simulink model "Szakdoga"  (R2018a)
settings: Solver=ode23s  StartTime=0.0  StopTime=6  RelTol=1e-3
values from neighbouring files (symbols this model uses):
  alp1 = (m1*lc1^2) + (m2*(l1^2+lc2^2)+I1+I2)    (= 1.6375)    [variables.m]
  alp2 = m2*l1*lc2    (= 0.4)    [variables.m]
  alp3 = (m2*lc2^2) + I2    (= 0.216667)    [variables.m]
undefined symbols (not defined in the file or in its folder): DiscIntNeverNeededParam
libraries: nesl_utility x9, sm_lib x8, simulink x6
settings Model: Creator=cloud  LastModifiedBy=cloud

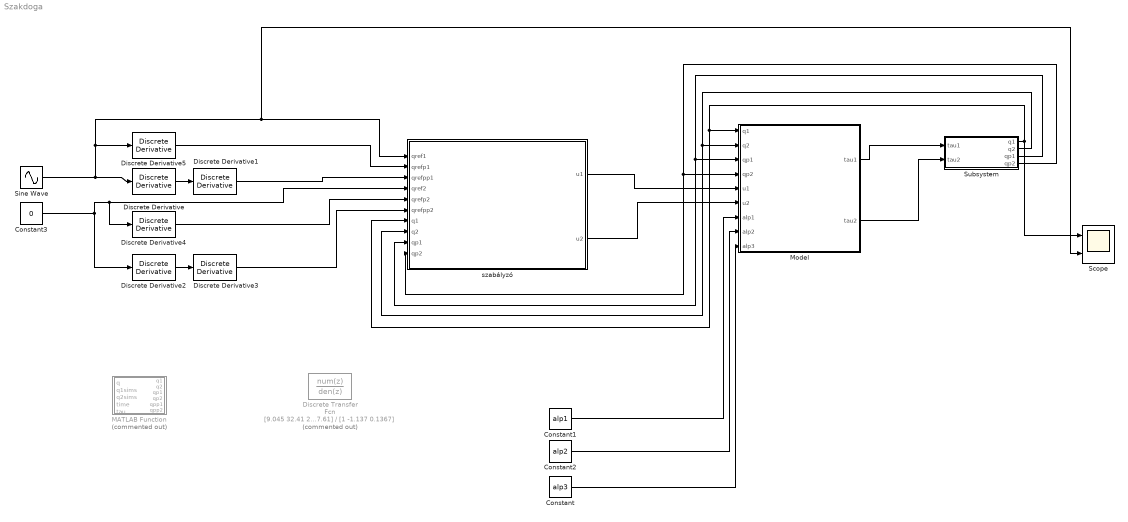
== system Szakdoga ==
  Constant : Constant  Value=alp3
  Constant1 : Constant  Value=alp1
  Constant2 : Constant  Value=alp2
  Constant3 : Constant  Value=0
  Discrete Transfer Fcn : DiscreteTransferFcn  Commented=on  Numerator=[9.045 32.41 27.61]  Denominator=[1 -1.137 0.1367]
  Discrete Derivative{,1..5} (6 alike) : simulink/Discrete/Discrete Derivative  gainval=1.0  ICPrevScaledInput=0.0  OutMin=[]  OutMax=[]  OutDataType=fixdt(1, 16)  OutScaling=2^-10  DoSatur=off
  MATLAB Function : MATLAB Function  Commented=on  TreatAsAtomicUnit=on
  Model : MATLAB Function  TreatAsAtomicUnit=on
  Scope : Scope  NumInputPorts=2
  Sine Wave : Sin  Amplitude=pi/2  Bias=pi/2  Frequency=1.5  SampleTime=0
  Subsystem : Subsystem
  szabályzó : Subsystem
  wires:
  Model/2(tau2) -> Subsystem/2(tau2)
  Model/1(tau1) -> Subsystem/1(tau1)
  Subsystem/2(q2) -> Model/2(q2), szabályzó/8(q2)
  Subsystem/3(qp1) -> Model/3(qp1), szabályzó/9(qp1)
  Subsystem/4(qp2) -> szabályzó/10(qp2), Model/4(qp2)
  Sine Wave/1 -> Discrete Derivative/1, Discrete Derivative5/1, Scope/2, szabályzó/1(qref1)
  Constant3/1 -> szabályzó/4(qref2), Discrete Derivative4/1, Discrete Derivative2/1
  Constant/1 -> Model/9(alp3)
  Constant2/1 -> Model/8(alp2)
  Constant1/1 -> Model/7(alp1)
  Discrete Derivative/1 -> Discrete Derivative1/1
  Discrete Derivative5/1 -> szabályzó/2(qrefp1)
  Discrete Derivative1/1 -> szabályzó/3(qrefpp1)
  Discrete Derivative4/1 -> szabályzó/5(qrefp2)
  szabályzó/1(u1) -> Model/5(u1)
  szabályzó/2(u2) -> Model/6(u2)
  Subsystem/1("q1 ") -> szabályzó/7(q1), Model/1(q1), Scope/1
  Discrete Derivative2/1 -> Discrete Derivative3/1
  Discrete Derivative3/1 -> szabályzó/6(qrefpp2)

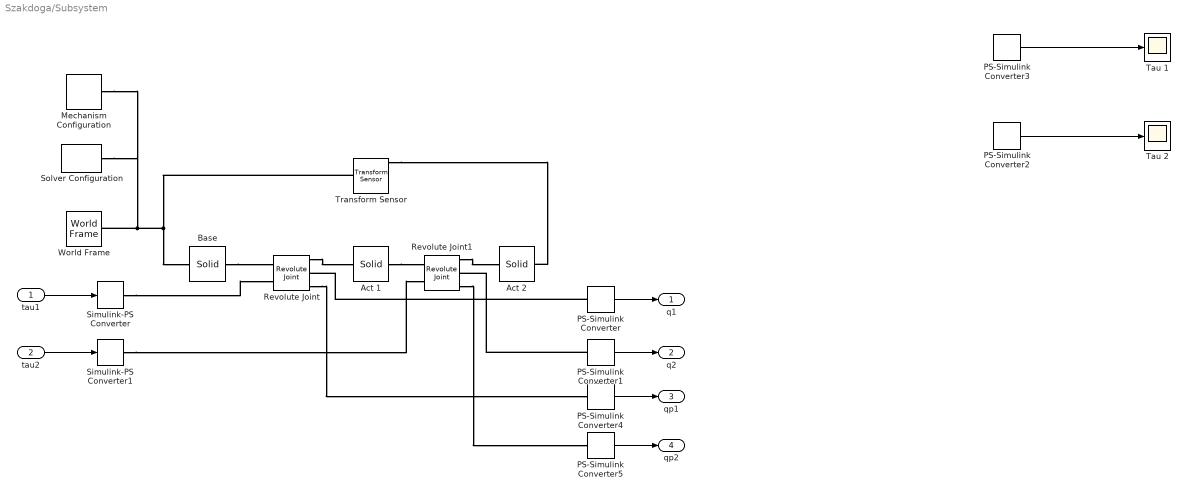
== system Szakdoga/Subsystem ==
  tau1 : Inport
  tau2 : Inport  Port=2
  Act 1 : sm_lib/Body Elements/Solid  InertiaType=CalculateFromGeometry  Mass=1  MassUnits=kg  CenterOfMass=[0 0 0]  CenterOfMassUnits=m  MomentsOfInertia=[1 1 1]  MomentsOfInertiaUnits=kg*m^2  ProductsOfInertia=[0 0 0]  ProductsOfInertiaUnits=kg*m^2  DensityBased=on  Density=1000  DensityUnits=kg/m^3  DoExposeReferenceFrame=off  SerializedFrames=<Frames><Frame><Id>Frame1</Id><Value><Name>F1</Name><Origin><Source>GeometricFeature</Source><FeatureName>-y -z curve</FeatureName></Origin><PrimaryAxis><DefinedDirection>+Z</DefinedDirection><Source>ReferenceFrame</Source><SourceDirection>+Z</SourceDirection><FeatureName></FeatureName></PrimaryAxis><SecondaryAxis><DefinedDirection>+X</DefinedDirection><Source>ReferenceFrame</Source><SourceDirection>+X</SourceDirection><FeatureName></FeatureName></SecondaryAxis></Value></Frame><Frame><Id>Frame2</Id><Value><Name>F2</Name><Origin><Source>GeometricFeature</Source><FeatureName>+y -z curve</FeatureName></Origin><PrimaryAxis><DefinedDirection>+Z</DefinedDirection><Source>ReferenceFrame</Source><SourceDirection>+Z</SourceDirection><FeatureName></FeatureName></PrimaryAxis><SecondaryAxis><DefinedDirection>+X</DefinedDirection><Source>ReferenceFrame</Source><SourceDirection>+X</SourceDirection><FeatureName></FeatureName></SecondaryAxis></Value></Frame></Frames>  GraphicType=FromGeometry  MarkerShape=Sphere  MarkerSize=10  GraphicVisPropType=SimpleVisualProperties  GraphicDiffuseColor=[0.5 0.5 0.5]  GraphicSpecularColor=[0.5 0.5 0.5 1.0]  GraphicAmbientColor=[0.15 0.15 0.15 1.0]  GraphicEmissiveColor=[0.0 0.0 0.0 1.0]  GraphicShininess=75  GraphicOpacity=1.0  GeometryShape=Brick  RectangleSize=[1 1]  RectangleSizeUnits=m  BrickDimensions=[0.1 0.5 0.1]  BrickDimensionUnits=m  CylinderRadius=1  CylinderRadiusUnits=m  CylinderLength=1  CylinderLengthUnits=m  SphereRadius=1  SphereRadiusUnits=m  EllipsoidRadii=[1 1 1]  EllipsoidRadiiUnits=m  ExtrusionCrossSection=[1 1; -1 1; -1 -1; 1 -1]  ExtrusionCrossSectionUnits=m  ExtrusionLength=1  ExtrusionLengthUnits=m  PolygonNumSides=3  PolygonOuterRadius=1  PolygonOuterRadiusUnits=m  ExtGeomFileType=STEP  ExtGeomFileUnits=m  RevolutionCrossSection=[1 1; 1 -1; 2 -1; 2 1]  RevolutionCrossSectionUnits=m  RevolutionExtent=Full  RevolutionAngle=180  RevolutionAngleUnits=deg
  Act 2 : sm_lib/Body Elements/Solid  InertiaType=CalculateFromGeometry  Mass=1  MassUnits=kg  CenterOfMass=[0 0 0]  CenterOfMassUnits=m  MomentsOfInertia=[1 1 1]  MomentsOfInertiaUnits=kg*m^2  ProductsOfInertia=[0 0 0]  ProductsOfInertiaUnits=kg*m^2  DensityBased=on  Density=1000  DensityUnits=kg/m^3  DoExposeReferenceFrame=off  SerializedFrames=<Frames><Frame><Id>Frame1</Id><Value><Name>F1</Name><Origin><Source>GeometricFeature</Source><FeatureName>-y +z curve</FeatureName></Origin><PrimaryAxis><DefinedDirection>+Z</DefinedDirection><Source>ReferenceFrame</Source><SourceDirection>+Z</SourceDirection><FeatureName></FeatureName></PrimaryAxis><SecondaryAxis><DefinedDirection>+X</DefinedDirection><Source>ReferenceFrame</Source><SourceDirection>+X</SourceDirection><FeatureName></FeatureName></SecondaryAxis></Value></Frame><Frame><Id>Frame2</Id><Value><Name>F2</Name><Origin><Source>GeometricFeature</Source><FeatureName>+y surface</FeatureName></Origin><PrimaryAxis><DefinedDirection>+Z</DefinedDirection><Source>ReferenceFrame</Source><SourceDirection>+Z</SourceDirection><FeatureName></FeatureName></PrimaryAxis><SecondaryAxis><DefinedDirection>+X</DefinedDirection><Source>ReferenceFrame</Source><SourceDirection>+X</SourceDirection><FeatureName></FeatureName></SecondaryAxis></Value></Frame></Frames>  GraphicType=FromGeometry  MarkerShape=Sphere  MarkerSize=10  GraphicVisPropType=SimpleVisualProperties  GraphicDiffuseColor=[0.5 0.5 0.5]  GraphicSpecularColor=[0.5 0.5 0.5 1.0]  GraphicAmbientColor=[0.15 0.15 0.15 1.0]  GraphicEmissiveColor=[0.0 0.0 0.0 1.0]  GraphicShininess=75  GraphicOpacity=1.0  GeometryShape=Brick  RectangleSize=[1 1]  RectangleSizeUnits=m  BrickDimensions=[0.1 0.4 0.1]  BrickDimensionUnits=m  CylinderRadius=1  CylinderRadiusUnits=m  CylinderLength=1  CylinderLengthUnits=m  SphereRadius=1  SphereRadiusUnits=m  EllipsoidRadii=[1 1 1]  EllipsoidRadiiUnits=m  ExtrusionCrossSection=[1 1; -1 1; -1 -1; 1 -1]  ExtrusionCrossSectionUnits=m  ExtrusionLength=1  ExtrusionLengthUnits=m  PolygonNumSides=3  PolygonOuterRadius=1  PolygonOuterRadiusUnits=m  ExtGeomFileType=STEP  ExtGeomFileUnits=m  RevolutionCrossSection=[1 1; 1 -1; 2 -1; 2 1]  RevolutionCrossSectionUnits=m  RevolutionExtent=Full  RevolutionAngle=180  RevolutionAngleUnits=deg
  Base : sm_lib/Body Elements/Solid  InertiaType=CalculateFromGeometry  Mass=1  MassUnits=kg  CenterOfMass=[0 0 0]  CenterOfMassUnits=m  MomentsOfInertia=[1 1 1]  MomentsOfInertiaUnits=kg*m^2  ProductsOfInertia=[0 0 0]  ProductsOfInertiaUnits=kg*m^2  DensityBased=on  Density=1000  DensityUnits=kg/m^3  DoExposeReferenceFrame=on  SerializedFrames=<Frames><Frame><Id>Frame1</Id><Value><Name>F1</Name><Origin><Source>GeometricFeature</Source><FeatureName>top surface</FeatureName></Origin><PrimaryAxis><DefinedDirection>+Z</DefinedDirection><Source>ReferenceFrame</Source><SourceDirection>+Z</SourceDirection><FeatureName></FeatureName></PrimaryAxis><SecondaryAxis><DefinedDirection>+X</DefinedDirection><Source>ReferenceFrame</Source><SourceDirection>-Y</SourceDirection><FeatureName></FeatureName></SecondaryAxis></Value></Frame></Frames>  GraphicType=FromGeometry  MarkerShape=Sphere  MarkerSize=10  GraphicVisPropType=SimpleVisualProperties  GraphicDiffuseColor=[0.5 0.5 0.5]  GraphicSpecularColor=[0.5 0.5 0.5 1.0]  GraphicAmbientColor=[0.15 0.15 0.15 1.0]  GraphicEmissiveColor=[0.0 0.0 0.0 1.0]  GraphicShininess=75  GraphicOpacity=1.0  GeometryShape=Cylinder  RectangleSize=[1 1]  RectangleSizeUnits=m  BrickDimensions=[1 1 1]  BrickDimensionUnits=m  CylinderRadius=0.07  CylinderRadiusUnits=m  CylinderLength=0.1  CylinderLengthUnits=m  SphereRadius=1  SphereRadiusUnits=m  EllipsoidRadii=[1 1 1]  EllipsoidRadiiUnits=m  ExtrusionCrossSection=[1 1; -1 1; -1 -1; 1 -1]  ExtrusionCrossSectionUnits=m  ExtrusionLength=1  ExtrusionLengthUnits=m  PolygonNumSides=3  PolygonOuterRadius=1  PolygonOuterRadiusUnits=m  ExtGeomFileType=STEP  ExtGeomFileUnits=m  RevolutionCrossSection=[1 1; 1 -1; 2 -1; 2 1]  RevolutionCrossSectionUnits=m  RevolutionExtent=Full  RevolutionAngle=180  RevolutionAngleUnits=deg
  Mechanism Configuration : sm_lib/Utilities/Mechanism Configuration  UniformGravity=Constant  GravityVector=[0 0 -9.80665]  GravityUnits=m/s^2  LinearizationDelta=0.001
  PS-Simulink Converter{,1..5} (6 alike) : nesl_utility/PS-Simulink Converter  PhysicalDomain=network_engine_domain  SubClassName=ps_output  LeftPortType=input  RightPortType=output  PseudoPeriodic=off  Frequencies=[]  Unit=1  AffineConversion=off
  Revolute Joint : sm_lib/Joints/Revolute Joint  SenseConstraintForce=off  SenseConstraintForceX=off  SenseConstraintForceY=off  SenseConstraintForceZ=off  SenseConstraintTorque=off  SenseConstraintTorqueX=off  SenseConstraintTorqueY=off  SenseConstraintTorqueZ=off  SenseTotalForce=off  SenseTotalForceX=off  SenseTotalForceY=off  SenseTotalForceZ=off  SenseTotalTorque=off  SenseTotalTorqueX=off  SenseTotalTorqueY=off  SenseTotalTorqueZ=off  CompositeWrenchDir=FollowerOnBase  CompositeWrenchFrame=BaseFrame  EquilibriumPosition=0  EquilibriumPositionUnits=deg  SpringStiffness=0  SpringStiffnessUnits=N*m/deg  DampingCoefficient=0  DampingCoefficientUnits=N*m/(deg/s)  TorqueActuationMode=InputTorque  MotionActuationMode=ComputedMotion  SensePosition=on  SenseVelocity=on  SenseAcceleration=off  SenseTorqueForce=off  PositionTargetSpecify=off  PositionTargetPriority=High  PositionTargetValue=0  PositionTargetValueUnits=deg  VelocityTargetSpecify=off  VelocityTargetPriority=High  VelocityTargetValue=0  VelocityTargetValueUnits=deg/s
  Revolute Joint1 : sm_lib/Joints/Revolute Joint  SenseConstraintForce=off  SenseConstraintForceX=off  SenseConstraintForceY=off  SenseConstraintForceZ=off  SenseConstraintTorque=off  SenseConstraintTorqueX=off  SenseConstraintTorqueY=off  SenseConstraintTorqueZ=off  SenseTotalForce=off  SenseTotalForceX=off  SenseTotalForceY=off  SenseTotalForceZ=off  SenseTotalTorque=off  SenseTotalTorqueX=off  SenseTotalTorqueY=off  SenseTotalTorqueZ=off  CompositeWrenchDir=FollowerOnBase  CompositeWrenchFrame=BaseFrame  EquilibriumPosition=0  EquilibriumPositionUnits=deg  SpringStiffness=0  SpringStiffnessUnits=N*m/deg  DampingCoefficient=0  DampingCoefficientUnits=N*m/(deg/s)  TorqueActuationMode=InputTorque  MotionActuationMode=ComputedMotion  SensePosition=on  SenseVelocity=on  SenseAcceleration=off  SenseTorqueForce=off  PositionTargetSpecify=off  PositionTargetPriority=High  PositionTargetValue=0  PositionTargetValueUnits=deg  VelocityTargetSpecify=off  VelocityTargetPriority=High  VelocityTargetValue=0  VelocityTargetValueUnits=deg/s
  Simulink-PS Converter : nesl_utility/Simulink-PS Converter  PhysicalDomain=network_engine_domain  SubClassName=ps_input  LeftPortType=input  RightPortType=output  PseudoPeriodic=off  Frequencies=[]  NoiseDistribution=none  NoiseParameters=[]  Unit=1  AffineConversion=off  FilteringAndDerivatives=filter  SimscapeFilterOrder=2  InputFilterTimeConstant=0.001  UdotUserProvided=0
  Simulink-PS Converter1 : nesl_utility/Simulink-PS Converter  PhysicalDomain=network_engine_domain  SubClassName=ps_input  LeftPortType=input  RightPortType=output  PseudoPeriodic=off  Frequencies=[]  NoiseDistribution=none  NoiseParameters=[]  Unit=1  AffineConversion=off  FilteringAndDerivatives=filter  SimscapeFilterOrder=2  InputFilterTimeConstant=0.001  UdotUserProvided=0
  Solver Configuration : nesl_utility/Solver Configuration  PhysicalDomain=network_engine_domain  SubClassName=solver  LeftPortType=input  RightPortType=generic  Tones=[]  Harmonics=[]  SimulateNoise=off  Profile=off  UseLocalSampling=off  EnableSwitchedLinearOptims=on  FrequencyDomain=off  UseCCode=off  RelTol=0.001  AbsTol=1e-06  MinStep=1e-09  ToWorkspace=off  RevertToSquareIcSolve=off  NumHomotopyIterations=100  PhasorMode=off  PhasorModeNumHarmonics=1  DoDC=off  ResidualTolerance=1e-09  UseLocalSolver=off  LocalSolverChoice=NE_BACKWARD_EULER_ADVANCER  LocalSolverSampleTime=0.001  DoFixedCost=off  MaxNonlinIter=3  MaxModeIter=2  LinearAlgebra=Sparse  EquationFormulation=NE_TIME_EF  DelaysMemoryBudget=1024  AutomaticFiltering=on  FilteringTimeConstant=0.001
  Tau 1 : Scope
  Tau 2 : Scope
  Transform Sensor : sm_lib/Frames and Transforms/Transform Sensor  MeasurementFrame=World  SenseAngle=off  SenseAxis=off  SenseAngle1=off  SenseAngle2=off  SenseAngle3=off  SenseQ=off  SenseR=off  SenseOmegaX=off  SenseOmegaY=off  SenseOmegaZ=off  SenseOmega1=off  SenseOmega2=off  SenseOmega3=off  SenseQDot=off  SenseRDot=off  SenseAlphaX=off  SenseAlphaY=off  SenseAlphaZ=off  SenseAlpha1=off  SenseAlpha2=off  SenseAlpha3=off  SenseQDDot=off  SenseRDDot=off  SenseX=on  SenseY=on  SenseZ=off  SenseRad=off  SenseAzim=off  SenseDist=off  SenseInc=off  SenseXDot=off  SenseYDot=off  SenseZDot=off  SenseRadDot=off  SenseAzimDot=off  SenseDistDot=off  SenseIncDot=off  SenseXDDot=off  SenseYDDot=off  SenseZDDot=off  SenseRadDDot=off  SenseAzimDDot=off  SenseDistDDot=off  SenseIncDDot=off
  World Frame : sm_lib/Frames and Transforms/World Frame
  "q1 " : Outport
  q2 : Outport  Port=2
  qp1 : Outport  Port=3
  qp2 : Outport  Port=4
  wires:
  tau1/1 -> Simulink-PS Converter/1
  tau2/1 -> Simulink-PS Converter1/1
  PS-Simulink Converter1/1 -> q2/1
  PS-Simulink Converter/1 -> "q1 "/1
  PS-Simulink Converter2/1 -> Tau 2/1
  PS-Simulink Converter3/1 -> Tau 1/1
  PS-Simulink Converter5/1 -> qp2/1
  PS-Simulink Converter4/1 -> qp1/1
  connections:
  Base/LConn1 -- Revolute Joint/LConn1
  Revolute Joint/RConn1 -- Act 1/LConn1
  Act 1/RConn1 -- Revolute Joint1/LConn1
  Revolute Joint1/RConn1 -- Act 2/LConn1
  Simulink-PS Converter/RConn1 -- Revolute Joint/LConn2
  Simulink-PS Converter1/RConn1 -- Revolute Joint1/LConn2
  PS-Simulink Converter1/LConn1 -- Revolute Joint1/RConn2
  PS-Simulink Converter/LConn1 -- Revolute Joint/RConn2
  Transform Sensor/LConn1 -- Mechanism Configuration/RConn1 -- Solver Configuration/RConn1 -- World Frame/RConn1 -- Base/RConn1
  Transform Sensor/RConn1 -- Act 2/RConn1
  Revolute Joint1/RConn3 -- PS-Simulink Converter5/LConn1
  Revolute Joint/RConn3 -- PS-Simulink Converter4/LConn1

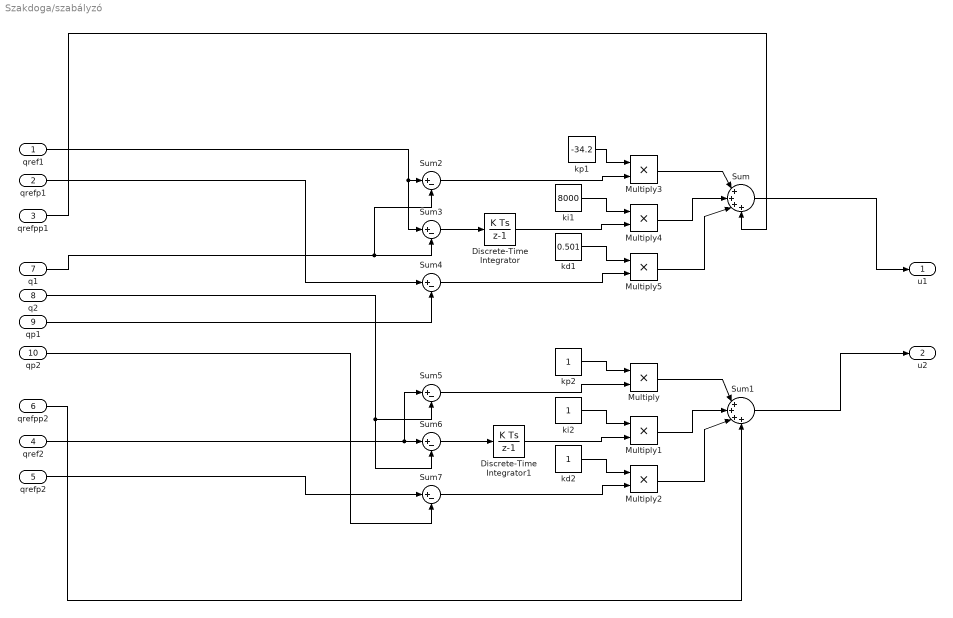
== system Szakdoga/szabályzó ==
  qref1 : Inport
  qrefp1 : Inport  Port=2
  qrefpp1 : Inport  Port=3
  qref2 : Inport  Port=4
  qrefp2 : Inport  Port=5
  qrefpp2 : Inport  Port=6
  q1 : Inport  Port=7
  q2 : Inport  Port=8
  qp1 : Inport  Port=9
  qp2 : Inport  Port=10
  Discrete-Time Integrator : DiscreteIntegrator  SampleTime=-1  ICPrevOutput=DiscIntNeverNeededParam  ICPrevScaledInput=DiscIntNeverNeededParam
  Discrete-Time Integrator1 : DiscreteIntegrator  SampleTime=0.01  ICPrevOutput=DiscIntNeverNeededParam  ICPrevScaledInput=DiscIntNeverNeededParam
  Multiply{,1..5} (6 alike) : Product
  Sum : Sum  Inputs=|++++
  Sum1 : Sum  Inputs=|++++
  Sum{2..7} (6 alike) : Sum  Inputs=|+-
  kd1 : Constant  Value=0.501
  kd2 : Constant
  ki1 : Constant  Value=8000
  ki2 : Constant
  kp1 : Constant  Value=-34.2
  kp2 : Constant
  u1 : Outport
  u2 : Outport  Port=2
  wires:
  qp2/1 -> Sum7/2
  q2/1 -> Sum5/2, Sum6/2
  Sum3/1 -> Discrete-Time Integrator/1
  Multiply4/1 -> Sum/2
  ki1/1 -> Multiply4/1
  Sum5/1 -> Multiply/2
  Multiply2/1 -> Sum1/3
  kd2/1 -> Multiply2/1
  Multiply/1 -> Sum1/1
  kd1/1 -> Multiply5/1
  Discrete-Time Integrator/1 -> Multiply4/2
  q1/1 -> Sum2/2, Sum3/2
  Multiply1/1 -> Sum1/2
  Sum2/1 -> Multiply3/2
  Multiply3/1 -> Sum/1
  qref2/1 -> Sum6/1, Sum5/1
  ki2/1 -> Multiply1/1
  Sum7/1 -> Multiply2/2
  qrefpp2/1 -> Sum1/4
  Discrete-Time Integrator1/1 -> Multiply1/2
  Sum6/1 -> Discrete-Time Integrator1/1
  qrefp2/1 -> Sum7/1
  qref1/1 -> Sum3/1, Sum2/1
  kp1/1 -> Multiply3/1
  Sum1/1 -> u2/1
  Multiply5/1 -> Sum/3
  qrefpp1/1 -> Sum/4
  Sum4/1 -> Multiply5/2
  kp2/1 -> Multiply/1
  qrefp1/1 -> Sum4/1
  qp1/1 -> Sum4/2
  Sum/1 -> u1/1

== matlab function Szakdoga/MATLAB Function ==
  data: q input; q1 output; q1sims input; q2sims input; time input; tau input; q2 output; qp1 output; qp2 output; qpp1 output; qpp2 output
function [q1,q2,qp1,qp2,qpp1,qpp2] = fcn(q, q1sims, q2sims, time, tau)

qc = q(1,:);
i=2;

while i<4
    %T = tau;
    
    %loading variables
    qbv= [q1sims,q2sims];
    qb = qc;
    qc = q(i,:);    
    
    %calculating travel time
    Ti = (qc-qb)/vmax;
    
    %calculating acceleraion time
    T = max(Ti,tau);
    
    %calculating speeds
    vbbv = (qb-qbv)/tau;
    vbc = (qc-qb)/T;
    
    %solving "a" variables
    a = C.'*y;
    t = -tau;
    
    while (t<T-tau)
        
        e
        
    end
    i=i+1;
end

x = tqpp2;
qpp2 = x;

== matlab function Szakdoga/Model ==
  data: q1 input; tau1 output; tau2 output; q2 input; qp1 input; qp2 input; u1 input; u2 input; alp1 input; alp2 input; alp3 input
function [tau1,tau2] = modell(q1,q2,qp1,qp2,u1,u2,alp1,alp2,alp3)

Y11 = u1;
Y12 = cos(q2)*(2*u1+u2)-sin(q2)*(qp1*qp2+qp1*qp2+qp2*qp2);
Y13 = u2;
Y21 = 0;
Y22 = cos(q2)*u1+sin(q2)*qp1*qp1;
Y23 = u1+u2;

tau1 = Y11*alp1+Y12*alp2+Y13*alp3;
tau2 = Y21*alp1+Y22*alp2+Y23*alp3;
x=tau2;
tau2 = x;
